simulink model "ref_sub_discretefilter"  (R2014b)
settings: Solver=ode45  StartTime=0.0  StopTime=10.0  RelTol=1e-3
settings Model: Creator=arnaud  LastModifiedBy=arnaud
settings DataIOCC: SaveFormat=Structure  SaveOutput=off  SaveTime=off

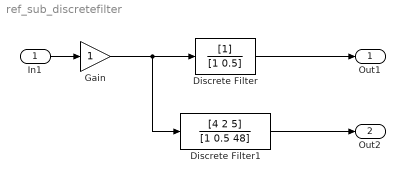
== system ref_sub_discretefilter ==
  In1 : Inport  OutDataTypeStr=double  PortDimensions=1  SampleTime=[1,0]
  Discrete Filter : DiscreteFilter  SampleTime=1
  Discrete Filter1 : DiscreteFilter  Numerator=[4 2 5]  Denominator=[1 0.5 48]  InitialStates=[1 0.9]  SampleTime=1
  Gain : Gain
  Out1 : Outport  OutDataTypeStr=double  PortDimensions=1  SampleTime=[1,0]
  Out2 : Outport  Port=2  OutDataTypeStr=double  PortDimensions=1  SampleTime=[1,0]
  wires:
  Discrete Filter/1 -> Out1/1
  Discrete Filter1/1 -> Out2/1
  In1/1 -> Gain/1
  Gain/1 -> Discrete Filter1/1, Discrete Filter/1
